simulink model "MatlabFunction1"  (R2017b)
settings: Solver=VariableStepAuto  StartTime=0.0  StopTime=10.0  RelTol=1e-3
settings Model: Creator=fconzelm  LastModifiedBy=hbourbou

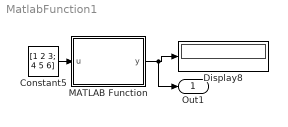
== system MatlabFunction1 ==
  Constant5 : Constant  Value=[1 2 3; 4 5 6]  OutDataTypeStr=int8
  Display8 : Display
  MATLAB Function : MATLAB Function  TreatAsAtomicUnit=on
  Out1 : Outport
  wires:
  Constant5/1 -> MATLAB Function/1(u)
  MATLAB Function/1(y) -> Out1/1, Display8/1

== matlab function MatlabFunction1/MATLAB Function ==
  data: u input; y output
function y = fcn(u)

y = sum(u);
